simulink model "eVTOL_System"  (R2024b)
settings: Solver=FixedStepAuto  StartTime=0.0  StopTime=inf  RelTol=1e-3
undefined symbols (not defined in the file): airspeed, Battery, BCE12, BCE_Set_init, BMS_Controller_State, C, Cell10_P, Cell11_P, Cell12_P, Cell13_P, Cell14_P, Cell15_P, Cell16_P, Cell17_P, Cell18_P, Cell19_P, Cell1_N, Cell1_P, Cell20_P, Cell21_P, Cell22_P, Cell23_P, Cell24_P, Cell2_P, Cell3_P, Cell4_P, Cell5_P, Cell6_P, Cell7_P, Cell8_P, Cell9_P, Charging_State, CityMission, control, controlParams, ControlSampleTime, CriticalTiltAngle, currentFactor, CV_Gain, ddx, ddy, ddz, Device_01, Device_02, DiscIntNeverNeededParam, dx, dy, dz, Earth, env, F, F28379D_ADC_MaxCount, F28379D_ADC_Vmax, FixedWingMission, flightState, Foc_Ki_IxTcpu, Foc_Ki_S, Foc_Kp_I, Foc_Kp_S, fractalcoef ... (+68)
libraries: fl_lib x1115, nesl_utility x617, slrealtimeethercatlib x217, simulink x130, canmsglib x101, speedgoatlib_IO611_obsolete x91, slpidlib x49, mcbcontrolslib x44, slrealtimeutilitieslib x35, speedgoatlib_hdlCoder_IO3xx x31, dspstat3 x24, mcbpositiondecoderlib x12
(part 7 of 31)

== system eVTOL_System/Flight Controller/Autopilot/Fixed Wing Controller/Fixed Wing Controller Simulation ==
  note: Attitude Controller
  note: Lateral Guidance
  note: Airspeed-Altitude Controller
  note: Visualization
  In Bus Element14 : Inport  PortName=States  Element=Xe
  In Bus Element32 : Inport  PortName=States  Element=Xe
  In Bus Element15 : Inport  PortName=States  Element=course
  In Bus Element17 : Inport  PortName=States  Element=pqr
  In Bus Element{5,22..23,29} (4 alike) : Inport  PortName=States  Element=airspeed
  In Bus Element19 : Inport  PortName=States  Element=ypr
  In Bus Element27 : Inport  PortName=States  Element=ypr
  In Bus Element16 : Inport  PortName=States  Element=gndspeed
  In Bus Element26 : Inport  PortName=States  Element=Euler
  In Bus Element20 : Inport  PortName=States  Element=Ve_ground
  In Bus Element11 : Inport  Port=2  PortName=Control Mode  Element=lateralGuidance
  In Bus Element12 : Inport  Port=2  PortName=Control Mode  Element=airspeedAltitude
  In Bus Element13 : Inport  Port=2  PortName=Control Mode  Element=attitude
  In Bus Element1 : Inport  Port=3  PortName=AAC SP  Element=airspeed
  In Bus Element24 : Inport  Port=3  PortName=AAC SP  Element=airspeed
  In Bus Element2 : Inport  Port=3  PortName=AAC SP  Element=altitude
  In Bus Element33 : Inport  Port=3  PortName=AAC SP  Element=altitude
  In Bus Element18 : Inport  Port=3  PortName=AAC SP  Element=L1
  In Bus Element21 : Inport  Port=3  PortName=AAC SP  Element=course
  In Bus Element3 : Inport  Port=3  PortName=AAC SP  Element=course
  In Bus Element4 : Inport  Port=4  PortName=FixedWingSP  Element=yaw
  In Bus Element28 : Inport  Port=4  PortName=FixedWingSP  Element=yaw
  In Bus Element9 : Inport  Port=4  PortName=FixedWingSP  Element=pitch
  In Bus Element10 : Inport  Port=4  PortName=FixedWingSP  Element=roll
  In Bus Element8 : Inport  Port=4  PortName=FixedWingSP  Element=airspeed
  In Bus Element : Inport  Port=5  PortName=AERT  Element=aileron
  In Bus Element6 : Inport  Port=5  PortName=AERT  Element=elevator
  In Bus Element7 : Inport  Port=5  PortName=AERT  Element=rudder
  AER from Path Manager : Subsystem  TreatAsAtomicUnit=on
  Actuator dT Merge : Merge
  Airspeed Altitude Scope : Scope  NumInputPorts=2
  Airspeed-Altitude Controller : Subsystem
  Attitude Controller : Subsystem
  Demux : Demux  Outputs=3
  Demux1 : Demux  Outputs=3
  Gain1 : Gain  Gain=-1
  Lateral Guidance Logic : Subsystem
  Merge : Merge
  Mux : Mux  Inputs=3
  Mux1 : Mux  Inputs=3
  Mux{2..6} (5 alike) : Mux  Inputs=2
  NOT : Logic  Operator=NOT  IconShape=distinctive  AllPortsSameDT=off  OutDataTypeStr=boolean
  NOT1 : Logic  Operator=NOT  IconShape=distinctive  AllPortsSameDT=off  OutDataTypeStr=boolean
  NOT2 : Logic  Operator=NOT  IconShape=distinctive  AllPortsSameDT=off  OutDataTypeStr=boolean
  Pitch SP Merge : Merge
  "Pitch, Airspeed SP from Controller" : Subsystem  TreatAsAtomicUnit=on
  Roll SP Merge : Merge
  Roll SP from Path Manager : Subsystem  TreatAsAtomicUnit=on
  Selector1 : Selector  InputPortWidth=3  IndexOptions=Index vector (dialog)  Indices=[3]  OutputSizes=1
  Subsystem2 : Subsystem
  YPR Scope : Scope  NumInputPorts=3
  Bus Element Out : Outport  PortName=Actuator  Element=dA
  Out Bus Element : Outport  PortName=Actuator  Element=dE
  Out Bus Element1 : Outport  PortName=Actuator  Element=dR
  Out Bus Element2 : Outport  PortName=Actuator  Element=dT
  wires:
  [PitchSP] -> Mux2/1  "ref"
  In Bus Element24/1 -> Mux5/1
  Mux6/1 -> Airspeed Altitude Scope/2  "Altitude Tracking"
  Pitch SP Merge/1 -> Mux/2, [PitchSP]
  Demux/2 -> Out Bus Element/1
  Airspeed-Altitude Controller/1(Pitch SP) -> Pitch SP Merge/1
  In Bus Element18/1 -> Lateral Guidance Logic/2(L1 Distance)
  In Bus Element1/1 -> Airspeed-Altitude Controller/1(Airspeed SP)
  In Bus Element17/1 -> Subsystem2/2(pqr)
  Demux1/3 -> Mux3/2
  Demux1/1 -> Mux4/2
  Actuator dT Merge/1 -> Out Bus Element2/1
  In Bus Element26/1 -> Subsystem2/1(Euler)
  In Bus Element11/1 -> Lateral Guidance Logic/Enable, NOT/1
  Subsystem2/1(Euler Rate) -> Attitude Controller/3(Ang Rate)
  In Bus Element13/1 -> NOT2/1, Attitude Controller/Enable
  In Bus Element3/1 -> Lateral Guidance Logic/1(Course SP)
  In Bus Element22/1 -> Attitude Controller/4(Airspeed)
  Demux/3 -> Out Bus Element1/1
  Roll SP from Path Manager/1(Out1) -> Roll SP Merge/2
  In Bus Element4/1 -> Mux/1
  In Bus Element14/1 -> Airspeed-Altitude Controller/5(xyz)
  In Bus Element15/1 -> Lateral Guidance Logic/3(course)
  In Bus Element27/1 -> Demux1/1
  In Bus Element6/1 -> Mux1/2
  Mux1/1 -> AER from Path Manager/1(In1)
  Airspeed-Altitude Controller/2(Throttle) -> Actuator dT Merge/1
  "Pitch, Airspeed SP from Controller"/1(Pitch SP) -> Pitch SP Merge/2
  In Bus Element16/1 -> Lateral Guidance Logic/4(gndspeed)
  "Pitch, Airspeed SP from Controller"/2(Throttle) -> Actuator dT Merge/2
  In Bus Element/1 -> Mux1/1
  In Bus Element2/1 -> Airspeed-Altitude Controller/2(Altitude SP)
  In Bus Element7/1 -> Mux1/3
  In Bus Element9/1 -> "Pitch, Airspeed SP from Controller"/1(Pitch SP In)
  Merge/1 -> Demux/1
  In Bus Element10/1 -> Roll SP from Path Manager/1(In1)
  Mux/1 -> Attitude Controller/1(YPR SP)
  Attitude Controller/1(AER) -> Merge/1
  Demux1/2 -> Mux2/2
  NOT1/1 -> "Pitch, Airspeed SP from Controller"/Enable
  Gain1/1 -> Mux6/2
  In Bus Element8/1 -> "Pitch, Airspeed SP from Controller"/2(Airspeed SP)
  In Bus Element33/1 -> Mux6/1  "REF"
  In Bus Element20/1 -> Airspeed-Altitude Controller/6(vxyz)
  Mux3/1 -> YPR Scope/3  "Roll Tracking"
  Selector1/1 -> Gain1/1
  In Bus Element19/1 -> Attitude Controller/2(ypr)
  In Bus Element32/1 -> Selector1/1
  NOT2/1 -> AER from Path Manager/Enable
  In Bus Element23/1 -> "Pitch, Airspeed SP from Controller"/3(Airspeed)
  In Bus Element29/1 -> Mux5/2
  Lateral Guidance Logic/1(Roll SP) -> Roll SP Merge/1
  In Bus Element28/1 -> Mux4/1
  NOT/1 -> Roll SP from Path Manager/Enable
  AER from Path Manager/1(Out1) -> Merge/2
  In Bus Element5/1 -> Airspeed-Altitude Controller/4(Airspeed)
  Demux/1 -> Bus Element Out/1
  In Bus Element21/1 -> Airspeed-Altitude Controller/3(Climb Rate SP)
  Mux5/1 -> Airspeed Altitude Scope/1  "Airspeed Tracking"
  Mux2/1 -> YPR Scope/2  "Pitch Tracking"
  Roll SP Merge/1 -> [RollSP], Mux/3
  In Bus Element12/1 -> Airspeed-Altitude Controller/Enable, NOT1/1
  [RollSP] -> Mux3/1  "ref"
  Mux4/1 -> YPR Scope/1  "Yaw Tracking"

== system eVTOL_System/Flight Controller/Autopilot/Fixed Wing Controller/Fixed Wing Controller Tuning ==
  note: Visualization
  note: Attitude Controller
  note: Airspeed-Altitude Controller
  note: Lateral Guidance
  In Bus Element14 : Inport  PortName=States  Element=Xe
  In Bus Element32 : Inport  PortName=States  Element=Xe
  In Bus Element15 : Inport  PortName=States  Element=course
  In Bus Element17 : Inport  PortName=States  Element=pqr
  In Bus Element{5,22..23,29} (4 alike) : Inport  PortName=States  Element=airspeed
  In Bus Element19 : Inport  PortName=States  Element=ypr
  In Bus Element27 : Inport  PortName=States  Element=ypr
  In Bus Element16 : Inport  PortName=States  Element=gndspeed
  In Bus Element26 : Inport  PortName=States  Element=Euler
  In Bus Element20 : Inport  PortName=States  Element=Ve_ground
  In Bus Element11 : Inport  Port=2  PortName=Control Mode  Element=lateralGuidance
  In Bus Element12 : Inport  Port=2  PortName=Control Mode  Element=airspeedAltitude
  In Bus Element13 : Inport  Port=2  PortName=Control Mode  Element=attitude
  In Bus Element1 : Inport  Port=3  PortName=AAC SP  Element=airspeed
  In Bus Element24 : Inport  Port=3  PortName=AAC SP  Element=airspeed
  In Bus Element2 : Inport  Port=3  PortName=AAC SP  Element=altitude
  In Bus Element33 : Inport  Port=3  PortName=AAC SP  Element=altitude
  In Bus Element18 : Inport  Port=3  PortName=AAC SP  Element=L1
  In Bus Element21 : Inport  Port=3  PortName=AAC SP  Element=course
  In Bus Element3 : Inport  Port=3  PortName=AAC SP  Element=course
  In Bus Element4 : Inport  Port=4  PortName=FixedWingSP  Element=yaw
  In Bus Element28 : Inport  Port=4  PortName=FixedWingSP  Element=yaw
  In Bus Element9 : Inport  Port=4  PortName=FixedWingSP  Element=pitch
  In Bus Element10 : Inport  Port=4  PortName=FixedWingSP  Element=roll
  In Bus Element8 : Inport  Port=4  PortName=FixedWingSP  Element=airspeed
  In Bus Element : Inport  Port=5  PortName=AERT  Element=aileron
  In Bus Element6 : Inport  Port=5  PortName=AERT  Element=elevator
  In Bus Element7 : Inport  Port=5  PortName=AERT  Element=rudder
  AER Switch : Switch  Criteria=u2 > Threshold  SaturateOnIntegerOverflow=off  InputSameDT=off
  AER from Path Manager : Subsystem  TreatAsAtomicUnit=on
  Actuator dT Switch : Switch  Criteria=u2 > Threshold  SaturateOnIntegerOverflow=off  InputSameDT=off
  Airspeed Altitude Scope : Scope  NumInputPorts=2
  Airspeed-Altitude Controller : Subsystem
  Attitude Controller : Subsystem
  Demux : Demux  Outputs=3
  Demux1 : Demux  Outputs=3
  Gain : Gain  Gain=-1
  Lateral Guidance Logic : Subsystem
  Mux : Mux  Inputs=3
  Mux1 : Mux  Inputs=3
  Mux{2..6} (5 alike) : Mux  Inputs=2
  NOT : Logic  Operator=NOT  IconShape=distinctive  AllPortsSameDT=off  OutDataTypeStr=boolean
  NOT1 : Logic  Operator=NOT  IconShape=distinctive  AllPortsSameDT=off  OutDataTypeStr=boolean
  NOT2 : Logic  Operator=NOT  IconShape=distinctive  AllPortsSameDT=off  OutDataTypeStr=boolean
  Pitch SP Switch : Switch  Criteria=u2 > Threshold  SaturateOnIntegerOverflow=off  InputSameDT=off
  "Pitch, Airspeed SP from Controller" : Subsystem  TreatAsAtomicUnit=on
  Roll SP Switch : Switch  Criteria=u2 > Threshold  SaturateOnIntegerOverflow=off  InputSameDT=off
  Roll SP from Path Manager : Subsystem  TreatAsAtomicUnit=on
  Selector1 : Selector  InputPortWidth=3  IndexOptions=Index vector (dialog)  Indices=[3]  OutputSizes=1
  Subsystem2 : Subsystem
  YPR Scope : Scope  NumInputPorts=3
  Bus Element Out : Outport  PortName=Actuator  Element=dA
  Out Bus Element : Outport  PortName=Actuator  Element=dE
  Out Bus Element1 : Outport  PortName=Actuator  Element=dR
  Out Bus Element2 : Outport  PortName=Actuator  Element=dT
  wires:
  Mux/1 -> Attitude Controller/1(YPR SP)
  Attitude Controller/1(AER) -> AER Switch/1
  AER Switch/1 -> Demux/1
  Demux/1 -> Bus Element Out/1
  NOT/1 -> Roll SP from Path Manager/Enable
  Lateral Guidance Logic/1(Roll SP) -> Roll SP Switch/1
  Roll SP from Path Manager/1(Out1) -> Roll SP Switch/3
  NOT1/1 -> "Pitch, Airspeed SP from Controller"/Enable
  In Bus Element8/1 -> "Pitch, Airspeed SP from Controller"/2(Airspeed SP)
  "Pitch, Airspeed SP from Controller"/1(Pitch SP) -> Pitch SP Switch/3
  Airspeed-Altitude Controller/2(Throttle) -> Actuator dT Switch/1
  "Pitch, Airspeed SP from Controller"/2(Throttle) -> Actuator dT Switch/3
  Mux1/1 -> AER from Path Manager/1(In1)
  AER from Path Manager/1(Out1) -> AER Switch/3
  NOT2/1 -> AER from Path Manager/Enable
  In Bus Element/1 -> Mux1/1
  In Bus Element6/1 -> Mux1/2
  In Bus Element7/1 -> Mux1/3
  In Bus Element9/1 -> "Pitch, Airspeed SP from Controller"/1(Pitch SP In)
  In Bus Element10/1 -> Roll SP from Path Manager/1(In1)
  In Bus Element11/1 -> Roll SP Switch/2, Lateral Guidance Logic/Enable, NOT/1
  In Bus Element18/1 -> Lateral Guidance Logic/2(L1 Distance)
  In Bus Element14/1 -> Airspeed-Altitude Controller/5(xyz)
  In Bus Element19/1 -> Attitude Controller/2(ypr)
  In Bus Element16/1 -> Lateral Guidance Logic/4(gndspeed)
  In Bus Element5/1 -> Airspeed-Altitude Controller/4(Airspeed)
  In Bus Element12/1 -> Actuator dT Switch/2, Pitch SP Switch/2, Airspeed-Altitude Controller/Enable, NOT1/1
  In Bus Element2/1 -> Airspeed-Altitude Controller/2(Altitude SP)
  Roll SP Switch/1 -> Mux/3, [RollSP]
  In Bus Element15/1 -> Lateral Guidance Logic/3(course)
  Demux/3 -> Out Bus Element1/1
  In Bus Element13/1 -> NOT2/1, AER Switch/2, Attitude Controller/Enable
  In Bus Element4/1 -> Mux/1
  In Bus Element22/1 -> Attitude Controller/4(Airspeed)
  In Bus Element3/1 -> Lateral Guidance Logic/1(Course SP)
  In Bus Element1/1 -> Airspeed-Altitude Controller/1(Airspeed SP)
  In Bus Element20/1 -> Airspeed-Altitude Controller/6(vxyz)
  In Bus Element21/1 -> Airspeed-Altitude Controller/3(Climb Rate SP)
  In Bus Element23/1 -> "Pitch, Airspeed SP from Controller"/3(Airspeed)
  In Bus Element27/1 -> Demux1/1
  Demux1/1 -> Mux4/2
  Demux1/2 -> Mux2/2
  Demux1/3 -> Mux3/2
  In Bus Element17/1 -> Subsystem2/2(pqr)
  In Bus Element26/1 -> Subsystem2/1(Euler)
  Subsystem2/1(Euler Rate) -> Attitude Controller/3(Ang Rate)
  Actuator dT Switch/1 -> Out Bus Element2/1
  Demux/2 -> Out Bus Element/1
  Pitch SP Switch/1 -> [PitchSP], Mux/2
  Airspeed-Altitude Controller/1(Pitch SP) -> Pitch SP Switch/1
  [PitchSP] -> Mux2/1  "ref"
  In Bus Element28/1 -> Mux4/1
  [RollSP] -> Mux3/1  "ref"
  Mux4/1 -> YPR Scope/1  "Yaw Tracking"
  Mux2/1 -> YPR Scope/2  "Pitch Tracking"
  Mux3/1 -> YPR Scope/3  "Roll Tracking"
  Mux5/1 -> Airspeed Altitude Scope/1  "Airspeed Tracking"
  Mux6/1 -> Airspeed Altitude Scope/2  "Altitude Tracking"
  In Bus Element24/1 -> Mux5/1
  In Bus Element29/1 -> Mux5/2
  In Bus Element32/1 -> Selector1/1
  Selector1/1 -> Gain/1
  Gain/1 -> Mux6/2
  In Bus Element33/1 -> Mux6/1  "REF"

== system eVTOL_System/Flight Controller/Autopilot/Multicopter Controller/Altitude Control ==
  note: Maintain altitude previously set when in transition
  Z ref : Inport
  States : Inport  Port=2
  InTransition : Inport  Port=3
  Bus Selector : BusSelector  OutputSignals=Xe,Ve
  Constant : Constant  Value=0
  Gain1 : Gain  Gain=controlParams.D_Z
  NOT : Logic  Operator=NOT  IconShape=distinctive  AllPortsSameDT=off  OutDataTypeStr=boolean
  PID Controller : slpidlib/PID Controller  Controller=P  Form=Parallel  TimeDomain=Discrete-time  UseExternalTs=off  SampleTime=-1  IntegratorMethod=Forward Euler  FilterMethod=Forward Euler  ControllerParametersSource=internal  P=controlParams.P_Z  I=controlParams.I_Z  UseKiTs=off  D=controlParams.D_Z  UseExternalDerivativeSource=off  N=controlParams.N_Z  UseFilter=on  TunerSelectOption=Transfer Function Based (PID Tuner App)  InitialConditionSource=internal  InitialConditionForIntegrator=0  InitialConditionForFilter=0  DifferentiatorICPrevScaledInput=0  ExternalReset=none  TrackingMode=off  Kt=1  LimitOutput=off  SatLimitsSource=internal  UpperSaturationLimit=inf  LowerSaturationLimit=-inf  LinearizeAsGain=on  AntiWindupMode=none  Kb=1  LimitIntegrator=off  UpperIntegratorSaturationLimit=inf  LowerIntegratorSaturationLimit=-inf  POutMin=[]  POutMax=[]  IOutMin=[]  IOutMax=[]  DOutMin=[]  DOutMax=[]  NOutMin=[]  NOutMax=[]  SumOutMin=[]  SumOutMax=[]  SaturationOutMin=[]  SaturationOutMax=[]  PParamMin=[]  PParamMax=[]  IParamMin=[]  IParamMax=[]  DParamMin=[]  DParamMax=[]  NParamMin=[]  NParamMax=[]  KbParamMin=[]  KbParamMax=[]  KtParamMin=[]  KtParamMax=[]  KbOutMin=[]  KbOutMax=[]  KtOutMin=[]  KtOutMax=[]  IntegratorOutMin=[]  IntegratorOutMax=[]  FilterOutMin=[]  FilterOutMax=[]  SumI1OutMin=[]  SumI1OutMax=[]  SumI2OutMin=[]  SumI2OutMax=[]  SumI3OutMin=[]  SumI3OutMax=[]  SumI4OutMin=[]  SumI4OutMax=[]  SumDOutMin=[]  SumDOutMax=[]  DifferentiatorOutMin=[]  DifferentiatorOutMax=[]  FilterDiffOutCoefMin=[]  FilterDiffOutCoefMax=[]  ReciprocalOutMin=[]  ReciprocalOutMax=[]  SumDenOutMin=[]  SumDenOutMax=[]  SumNumOutMin=[]  SumNumOutMax=[]  DivideOutMin=[]  DivideOutMax=[]  UdiffTsProdOutMin=[]  UdiffTsProdOutMax=[]  NTsProdOutMin=[]  NTsProdOutMax=[]  UintegralTsProdOutMin=[]  UintegralTsProdOutMax=[]  UngainTsProdOutMin=[]  UngainTsProdOutMax=[]  ClampingZeroOutDataTypeStr=Inherit: Inherit via back propagation  ClampingZeroOutMin=[]  ClampingZeroOutMax=[]  FilterDenConstantOutDataTypeStr=Inherit: Inherit via back propagation  FilterDenConstantOutMin=[]  FilterDenConstantOutMax=[]  PCopyOutDataTypeStr=Inherit: Inherit via back propagation  PCopyOutMin=[]  PCopyOutMax=[]  NCopyOutDataTypeStr=Inherit: Inherit via back propagation  NCopyOutMin=[]  NCopyOutMax=[]  IntegratorContinuousStateAttributes=''  IntegratorStateMustResolveToSignalObject=off  IntegratorRTWStateStorageClass=Auto  FilterContinuousStateAttributes=''  FilterStateMustResolveToSignalObject=off  FilterRTWStateStorageClass=Auto  ParallelPVariant=InternalParameters  IdealPVariant=Disabled  IVariant=Disabled  DVariant=Disabled  IntegratorVariant=Disabled  SatVariant=Disabled  AWVariant=Disabled  PCopyVariant=Disabled  TRVariant=Disabled  FdbkBlocksVariant=Forward  IdealPFdbkVariant=Disabled  SatFdbkVariant=Disabled  DerivativeFilterVariant=Disabled  NVariant=Disabled  NCopyVariant=Disabled_SignalSpec  FilterICVariant=Disabled  IntegratorICVariant=Disabled  ExternalResetVariant=Disabled  TRSumVariant=Passthrough  SumFdbkVariant=Disabled  SumVariant=Passthrough_P  TsampFilterVariant=InternalTs  TsampNgainVariant=Passthrough  TsampIntegralVariant=Disabled_SignalSpec  ExternalSaturationOutDataTypeStr=Inherit: Same as second input  DerivativeSourceVariant=Disabled  PreIntVariant=InternalPreInt
  PID Controller1 : slpidlib/PID Controller  Controller=PID  Form=Parallel  TimeDomain=Discrete-time  UseExternalTs=off  SampleTime=-1  IntegratorMethod=Forward Euler  FilterMethod=Forward Euler  ControllerParametersSource=internal  P=controlParams.P_VZ  I=controlParams.I_Z  UseKiTs=off  D=controlParams.D_VZ  UseExternalDerivativeSource=off  N=controlParams.N_VZ  UseFilter=on  TunerSelectOption=Transfer Function Based (PID Tuner App)  InitialConditionSource=internal  InitialConditionForIntegrator=0  InitialConditionForFilter=0  DifferentiatorICPrevScaledInput=0  ExternalReset=none  TrackingMode=off  Kt=1  LimitOutput=off  SatLimitsSource=internal  UpperSaturationLimit=inf  LowerSaturationLimit=-inf  LinearizeAsGain=on  AntiWindupMode=none  Kb=1  LimitIntegrator=off  UpperIntegratorSaturationLimit=inf  LowerIntegratorSaturationLimit=-inf  POutMin=[]  POutMax=[]  IOutMin=[]  IOutMax=[]  DOutMin=[]  DOutMax=[]  NOutMin=[]  NOutMax=[]  SumOutMin=[]  SumOutMax=[]  SaturationOutMin=[]  SaturationOutMax=[]  PParamMin=[]  PParamMax=[]  IParamMin=[]  IParamMax=[]  DParamMin=[]  DParamMax=[]  NParamMin=[]  NParamMax=[]  KbParamMin=[]  KbParamMax=[]  KtParamMin=[]  KtParamMax=[]  KbOutMin=[]  KbOutMax=[]  KtOutMin=[]  KtOutMax=[]  IntegratorOutMin=[]  IntegratorOutMax=[]  FilterOutMin=[]  FilterOutMax=[]  SumI1OutMin=[]  SumI1OutMax=[]  SumI2OutMin=[]  SumI2OutMax=[]  SumI3OutMin=[]  SumI3OutMax=[]  SumI4OutMin=[]  SumI4OutMax=[]  SumDOutMin=[]  SumDOutMax=[]  DifferentiatorOutMin=[]  DifferentiatorOutMax=[]  FilterDiffOutCoefMin=[]  FilterDiffOutCoefMax=[]  ReciprocalOutMin=[]  ReciprocalOutMax=[]  SumDenOutMin=[]  SumDenOutMax=[]  SumNumOutMin=[]  SumNumOutMax=[]  DivideOutMin=[]  DivideOutMax=[]  UdiffTsProdOutMin=[]  UdiffTsProdOutMax=[]  NTsProdOutMin=[]  NTsProdOutMax=[]  UintegralTsProdOutMin=[]  UintegralTsProdOutMax=[]  UngainTsProdOutMin=[]  UngainTsProdOutMax=[]  ClampingZeroOutDataTypeStr=Inherit: Inherit via back propagation  ClampingZeroOutMin=[]  ClampingZeroOutMax=[]  FilterDenConstantOutDataTypeStr=Inherit: Inherit via back propagation  FilterDenConstantOutMin=[]  FilterDenConstantOutMax=[]  PCopyOutDataTypeStr=Inherit: Inherit via back propagation  PCopyOutMin=[]  PCopyOutMax=[]  NCopyOutDataTypeStr=Inherit: Inherit via back propagation  NCopyOutMin=[]  NCopyOutMax=[]  IntegratorContinuousStateAttributes=''  IntegratorStateMustResolveToSignalObject=off  IntegratorRTWStateStorageClass=Auto  FilterContinuousStateAttributes=''  FilterStateMustResolveToSignalObject=off  FilterRTWStateStorageClass=Auto  ParallelPVariant=InternalParameters  IdealPVariant=Disabled  IVariant=InternalParameters  DVariant=InternalParameters  IntegratorVariant=Discrete  SatVariant=Disabled  AWVariant=Passthrough  PCopyVariant=Disabled  TRVariant=Disabled  FdbkBlocksVariant=Forward  IdealPFdbkVariant=Disabled  SatFdbkVariant=Disabled  DerivativeFilterVariant=ForwardEulerFilter  NVariant=InternalParameters  NCopyVariant=Disabled  FilterICVariant=InternalICsFilter  IntegratorICVariant=InternalICs  ExternalResetVariant=Disabled  TRSumVariant=Passthrough  SumFdbkVariant=Disabled  SumVariant=Sum_PID  TsampFilterVariant=InternalTs  TsampNgainVariant=Passthrough  TsampIntegralVariant=Disabled_SignalSpec  ExternalSaturationOutDataTypeStr=Inherit: Same as second input  DerivativeSourceVariant=ErrorSignal  PreIntVariant=InternalPreInt
  Rate Limiter : RateLimiter  FallingSlewLimit=-1000  SampleTimeMode=inherited
  Selector : Selector  InputPortWidth=3  IndexOptions=Index vector (dialog)  Indices=[3]  OutputSizes=1
  Selector1 : Selector  InputPortWidth=3  IndexOptions=Index vector (dialog)  Indices=[3]  OutputSizes=1
  Sum : Sum  Inputs=|+-
  Sum1 : Sum  Inputs=|+-
  Sum2 : Sum  Inputs=|++
  Sum3 : Sum  Inputs=|--
  Switch : Switch  Criteria=u2 > Threshold  SaturateOnIntegerOverflow=off  InputSameDT=off
  Triggered Subsystem : Subsystem  TreatAsAtomicUnit=on
  commanded thrust : Outport
  wires:
  Sum/1 -> PID Controller/1
  Z ref/1 -> Switch/1  "Manual"
  States/1 -> Bus Selector/1
  InTransition/1 -> NOT/1, Triggered Subsystem/Trigger
  Switch/1 -> Rate Limiter/1  "Output"
  NOT/1 -> Switch/2
  Triggered Subsystem/1(Reference) -> Switch/3  "Stable"
  Selector/1 -> Sum/2, Triggered Subsystem/1(AltHold)
  Bus Selector/1 -> Selector/1  "<Xe>"
  Bus Selector/2 -> Selector1/1  "<Ve>"
  PID Controller/1 -> Sum2/1
  Selector1/1 -> Sum1/2, Gain1/1
  Gain1/1 -> Sum3/2
  Sum2/1 -> Sum1/1
  Sum1/1 -> PID Controller1/1
  Rate Limiter/1 -> Sum/1
  Sum3/1 -> Sum2/2
  PID Controller1/1 -> commanded thrust/1
  Constant/1 -> Sum3/1

== system eVTOL_System/Flight Controller/Autopilot/Multicopter Controller/Attitude Control ==
  Ref Attitude : Inport
  States : Inport  Port=2
  inTransition : Inport  Port=3
  Attitude Control : Subsystem  VariantControl=AttitudeControl==0
  Derivative Gain : Subsystem  VariantControl=AttitudeControl==1
  Roll torque cmd : Outport
  Pitch torque Cmd : Outport  Port=2
  Yaw torque Cmd : Outport  Port=3

== system eVTOL_System/Flight Controller/Autopilot/Multicopter Controller/Attitude Stabilization ==
  note: Level Tiltrotor when in transition.
  Enable : EnablePort
  Constant : Constant  Value=0
  Constant1 : Constant  Value=0
  Tilt Cmd : Outport
  Roll Cmd : Outport  Port=2
  wires:
  Constant/1 -> Tilt Cmd/1
  Constant1/1 -> Roll Cmd/1

== system eVTOL_System/Flight Controller/Autopilot/Multicopter Controller/Horizontal Position Control ==
  note: Forward Motion is controlled using Tilt.
      | Lateral Motion occurs using roll.
  XRef : Inport
  YRef : Inport  Port=2
  States : Inport  Port=3
  Enable : EnablePort
  Saturation : Saturate  UpperLimit=0.4  LowerLimit=-0.4
  XY Controller : Subsystem
  Roll Cmd : Outport
  Tilt Cmd : Outport  Port=2
  wires:
  XRef/1 -> XY Controller/1(X_ref)
  YRef/1 -> XY Controller/2(Y_ref)
  States/1 -> XY Controller/3(States)
  XY Controller/1(Forward cmd) -> Tilt Cmd/1
  XY Controller/2(Sideward Cmd) -> Saturation/1
  Saturation/1 -> Roll Cmd/1

== system eVTOL_System/Flight Controller/Autopilot/Multicopter Controller/Organize Inputs ==
  forward command : Inport
  commanded phi torque : Inport  Port=2
  commanded theta torque : Inport  Port=3
  commanded psi torque : Inport  Port=4
  commanded thrust : Inport  Port=5
  Out Bus Element : Outport  PortName=MixerCommands  Element=w_phi
  Out Bus Element1 : Outport  PortName=MixerCommands  Element=w_theta
  Out Bus Element2 : Outport  PortName=MixerCommands  Element=l_psi
  Out Bus Element3 : Outport  PortName=MixerCommands  Element=w_z
  Out Bus Element4 : Outport  PortName=MixerCommands  Element=l_x
  tag scope: w_phi=global, w_psi=global, w_theta=global, w_tilt=global, w_z=global
  wires:
  commanded theta torque/1 -> Out Bus Element1/1, [w_theta]  "theta"
  commanded psi torque/1 -> Out Bus Element2/1, [w_psi]  "psi"
  commanded thrust/1 -> Out Bus Element3/1, [w_z]  "thrust"
  forward command/1 -> Out Bus Element4/1, [w_tilt]  "tilt"
  commanded phi torque/1 -> Out Bus Element/1, [w_phi]  "phi"

== system eVTOL_System/Flight Controller/Autopilot/Multicopter Controller/Subsystem ==
  inTransition : Inport
  States : Inport  Port=2
  Reference : Inport  Port=3
  Bus Selector : BusSelector  OutputSignals=ypr
  Bus Selector1 : BusSelector  OutputSignals=ypr,Euler
  NOT : Logic  Operator=NOT  IconShape=distinctive  AllPortsSameDT=off  OutDataTypeStr=boolean
  Scope{,1..3} (4 alike) : Scope
  Selector : Selector  InputPortWidth=3  IndexOptions=Index vector (dialog)  Indices=[1]  OutputSizes=1
  Switch : Switch  Criteria=u2 > Threshold  SaturateOnIntegerOverflow=off  InputSameDT=off
  Triggered Subsystem : Subsystem  TreatAsAtomicUnit=on
  Yaw Reference : Outport
  wires:
  inTransition/1 -> Triggered Subsystem/Trigger, NOT/1
  States/1 -> Bus Selector1/1, Bus Selector/1
  Bus Selector/1 -> Selector/1  "<ypr>"
  Selector/1 -> Triggered Subsystem/1(YawHold)
  NOT/1 -> Switch/2
  Triggered Subsystem/1(Reference) -> Switch/3, Scope1/1  "Stable"
  Switch/1 -> Scope/1, Yaw Reference/1
  Bus Selector1/1 -> Scope2/1  "<ypr>"
  Bus Selector1/2 -> Scope3/1  "<Euler>"
  Reference/1 -> Switch/1

== system eVTOL_System/Flight Controller/Autopilot/Tilt Scheduler/Back Transition Scheduler ==
  Tilt Schedule : Inport
  FlightMode : Inport  Port=2
  States : Inport  Port=3
  Add : Sum  Inputs=+-
  Bus Selector : BusSelector  OutputSignals=Vb
  Constant1 : Constant  Value=flightState.BackTransition
  Constant6 : Constant  Value=0
  Equal1 : RelationalOperator  Operator===  OutDataTypeStr=boolean  RndMeth=Simplest  InputSameDT=off
  Saturation : Saturate  UpperLimit=pi/4  LowerLimit=-pi/4
  Selector : Selector  InputPortWidth=3  IndexOptions=Index vector (dialog)  Indices=[1]  OutputSizes=1
  Switch2 : Switch  Threshold=1  SaturateOnIntegerOverflow=off  InputSameDT=off
  Vx Controller : slpidlib/PID Controller  Controller=P  Form=Parallel  TimeDomain=Discrete-time  UseExternalTs=off  SampleTime=0.005  IntegratorMethod=Forward Euler  FilterMethod=Forward Euler  ControllerParametersSource=internal  P=controlParams.P_BACK  I=0  UseKiTs=off  D=0.0379422021775223  UseExternalDerivativeSource=off  N=1.96946409823213  UseFilter=on  TunerSelectOption=Transfer Function Based (PID Tuner App)  InitialConditionSource=internal  InitialConditionForIntegrator=0  InitialConditionForFilter=0  DifferentiatorICPrevScaledInput=0  ExternalReset=none  TrackingMode=off  Kt=1  LimitOutput=off  SatLimitsSource=internal  UpperSaturationLimit=inf  LowerSaturationLimit=-inf  LinearizeAsGain=on  AntiWindupMode=none  Kb=1  LimitIntegrator=off  UpperIntegratorSaturationLimit=inf  LowerIntegratorSaturationLimit=-inf  POutMin=[]  POutMax=[]  IOutMin=[]  IOutMax=[]  DOutMin=[]  DOutMax=[]  NOutMin=[]  NOutMax=[]  SumOutMin=[]  SumOutMax=[]  SaturationOutMin=[]  SaturationOutMax=[]  PParamMin=[]  PParamMax=[]  IParamMin=[]  IParamMax=[]  DParamMin=[]  DParamMax=[]  NParamMin=[]  NParamMax=[]  KbParamMin=[]  KbParamMax=[]  KtParamMin=[]  KtParamMax=[]  KbOutMin=[]  KbOutMax=[]  KtOutMin=[]  KtOutMax=[]  IntegratorOutMin=[]  IntegratorOutMax=[]  FilterOutMin=[]  FilterOutMax=[]  SumI1OutMin=[]  SumI1OutMax=[]  SumI2OutMin=[]  SumI2OutMax=[]  SumI3OutMin=[]  SumI3OutMax=[]  SumI4OutMin=[]  SumI4OutMax=[]  SumDOutMin=[]  SumDOutMax=[]  DifferentiatorOutMin=[]  DifferentiatorOutMax=[]  FilterDiffOutCoefMin=[]  FilterDiffOutCoefMax=[]  ReciprocalOutMin=[]  ReciprocalOutMax=[]  SumDenOutMin=[]  SumDenOutMax=[]  SumNumOutMin=[]  SumNumOutMax=[]  DivideOutMin=[]  DivideOutMax=[]  UdiffTsProdOutMin=[]  UdiffTsProdOutMax=[]  NTsProdOutMin=[]  NTsProdOutMax=[]  UintegralTsProdOutMin=[]  UintegralTsProdOutMax=[]  UngainTsProdOutMin=[]  UngainTsProdOutMax=[]  ClampingZeroOutDataTypeStr=Inherit: Inherit via back propagation  ClampingZeroOutMin=[]  ClampingZeroOutMax=[]  FilterDenConstantOutDataTypeStr=Inherit: Inherit via back propagation  FilterDenConstantOutMin=[]  FilterDenConstantOutMax=[]  PCopyOutDataTypeStr=Inherit: Inherit via back propagation  PCopyOutMin=[]  PCopyOutMax=[]  NCopyOutDataTypeStr=Inherit: Inherit via back propagation  NCopyOutMin=[]  NCopyOutMax=[]  IntegratorContinuousStateAttributes=''  IntegratorStateMustResolveToSignalObject=off  IntegratorRTWStateStorageClass=Auto  FilterContinuousStateAttributes=''  FilterStateMustResolveToSignalObject=off  FilterRTWStateStorageClass=Auto  ParallelPVariant=InternalParameters  IdealPVariant=Disabled  IVariant=Disabled  DVariant=Disabled  IntegratorVariant=Disabled  SatVariant=Disabled  AWVariant=Disabled  PCopyVariant=Disabled  TRVariant=Disabled  FdbkBlocksVariant=Forward  IdealPFdbkVariant=Disabled  SatFdbkVariant=Disabled  DerivativeFilterVariant=Disabled  NVariant=Disabled  NCopyVariant=Disabled_SignalSpec  FilterICVariant=Disabled  IntegratorICVariant=Disabled  ExternalResetVariant=Disabled  TRSumVariant=Passthrough  SumFdbkVariant=Disabled  SumVariant=Passthrough_P  TsampFilterVariant=InternalTs  TsampNgainVariant=Passthrough  TsampIntegralVariant=Disabled_SignalSpec  ExternalSaturationOutDataTypeStr=Inherit: Same as second input  DerivativeSourceVariant=Disabled  PreIntVariant=InternalPreInt
  TiltAngle : Outport
  wires:
  States/1 -> Bus Selector/1
  Add/1 -> Vx Controller/1
  Equal1/1 -> Switch2/2
  Bus Selector/1 -> Selector/1  "<Vb>"
  FlightMode/1 -> Equal1/1
  Constant1/1 -> Equal1/2
  Constant6/1 -> Add/1
  Selector/1 -> Add/2
  Vx Controller/1 -> Saturation/1
  Saturation/1 -> Switch2/1
  Tilt Schedule/1 -> Switch2/3
  Switch2/1 -> TiltAngle/1

== system eVTOL_System/Flight Controller/Autopilot/Tilt Scheduler/Forward Transition Scheduler ==
  FlightMode : Inport
  Constant : Constant  Value=pi/2
  Constant2 : Constant  Value=0
  Constant3 : Constant  Value=CriticalTiltAngle
  Constant4 : Constant  Value=flightState.Transition
  Constant5 : Constant  Value=TiltScheduleRate
  Equal : RelationalOperator  Operator===  OutDataTypeStr=boolean  RndMeth=Simplest  InputSameDT=off
  Integrator : Integrator  ExternalReset=either  LimitOutput=on  UpperSaturationLimit=Inf  LowerSaturationLimit=0
  LessThanOrEqual : RelationalOperator  Operator=<=  OutDataTypeStr=boolean  RndMeth=Simplest  InputSameDT=off
  Switch : Switch  Criteria=u2 > Threshold  SaturateOnIntegerOverflow=off  InputSameDT=off
  Switch1 : Switch  Criteria=u2 > Threshold  SaturateOnIntegerOverflow=off  InputSameDT=off
  FlightState : Outport
  Tilt Schedule : Outport  Port=2
  tag scope: ModeFlag=global
  wires:
  FlightMode/1 -> FlightState/1, Equal/2
  [ModeFlag] -> Switch1/2, Integrator/2
  Integrator/1 -> Switch/1, LessThanOrEqual/1
  LessThanOrEqual/1 -> Switch/2
  Equal/1 -> [ModeFlag]
  Constant3/1 -> LessThanOrEqual/2
  Switch1/1 -> Integrator/1
  Constant5/1 -> Switch1/1
  Constant2/1 -> Switch1/3
  Constant4/1 -> Equal/1
  Constant/1 -> Switch/3
  Switch/1 -> Tilt Schedule/1

== system eVTOL_System/Flight Controller/Estimator/Estimation Filter/Airspeed Filter ==
  DiffPress : Inport
  rho : Inport  Port=2
  Constant : Constant  Value=0.5
  Divide : Product  Inputs=*/
  Product : Product
  Sqrt : Sqrt
  airspeed : Outport
  wires:
  Constant/1 -> Product/2
  rho/1 -> Product/1
  Product/1 -> Divide/2
  DiffPress/1 -> Divide/1
  Divide/1 -> Sqrt/1
  Sqrt/1 -> airspeed/1

== system eVTOL_System/Flight Controller/Estimator/Estimation Filter/LLA2Local ==
  LLA : Inport
  Constant1 : Constant  Value=0
  Demux1 : Demux  Outputs=2
  LLA to Flat Earth1 : aerolibtransform2/LLA to Flat Earth  units=Metric (MKS)  ptype=Earth (WGS84)  F=1/298.257223563  R=6378137  refPosPort=off  LL0=[0 0]  psi=0
  Xe : Outport
  wires:
  Constant1/1 -> LLA to Flat Earth1/3
  Demux1/1 -> LLA to Flat Earth1/1
  Demux1/2 -> LLA to Flat Earth1/2
  LLA to Flat Earth1/1 -> Xe/1  "Xe"
  LLA/1 -> Demux1/1

== system eVTOL_System/Flight Controller/Ground Control Station/Get Flight Mission/noQGC ==
  note: uavPathManagerBus type
  No Mission : Constant  Value=struct('mode',0,'position',[0 0 0]','params',[0;0;0;0]);  OutDataTypeStr=Bus: doubleUavPathManager
  Variant Source : VariantSource
  Waypoints : Constant  Value=FixedWingMission  OutDataTypeStr=Bus: doubleUavPathManager  SampleTime=-1
  Waypoints1 : Constant  Value=HoverMission  OutDataTypeStr=Bus: doubleUavPathManager  SampleTime=-1
  Waypoints2 : Constant  Value=TransitionMission  OutDataTypeStr=Bus: doubleUavPathManager  SampleTime=-1
  Waypoints3 : Constant  Value=CityMission  OutDataTypeStr=Bus: doubleUavPathManager  SampleTime=-1
  Mission : Outport
  wires:
  Waypoints/1 -> Variant Source/2
  Waypoints1/1 -> Variant Source/3
  Variant Source/1 -> Mission/1
  Waypoints2/1 -> Variant Source/4
  No Mission/1 -> Variant Source/1
  Waypoints3/1 -> Variant Source/5

== system eVTOL_System/Flight Controller/Guidance Test Bench/ControlType/Guidance Testbench ==
  Global Mission : Inport
  Aircraft States : Inport  Port=2
  Control Rate Transition : Subsystem
  Guidance Logic : Subsystem  VariantControl=guidanceType==1
  HoverCmds : Outport
  FixedWingSP : Outport  Port=2
  AACSP : Outport  Port=3
  ctrlMode : Outport  Port=4
  FlightMode : Outport  Port=5
  wires:
  Aircraft States/1 -> Guidance Logic/1(UAVState)
  Global Mission/1 -> Guidance Logic/2(GCSCommands)
  Guidance Logic/1(HoverGuidance) -> Control Rate Transition/1("1 ")
  Guidance Logic/2(FixedWingSP) -> Control Rate Transition/2(In2)
  Guidance Logic/3(AACSP) -> Control Rate Transition/3(In3)
  Guidance Logic/4(ctrlMode) -> Control Rate Transition/4(In4)
  Guidance Logic/5(FlightMode) -> Control Rate Transition/5(In5)
  Control Rate Transition/1(Out1) -> HoverCmds/1
  Control Rate Transition/2(Out2) -> FixedWingSP/1
  Control Rate Transition/3(Out3) -> AACSP/1
  Control Rate Transition/4(Out4) -> ctrlMode/1
  Control Rate Transition/5(Out5) -> FlightMode/1

== system eVTOL_System/Flight Controller/Guidance Test Bench/ControlType/Manual Control ==
  note: Change these parameters during simulation when using manual testbench mode.
  note: Commanded Altitude (m)
  note: Commanded Y (m)
  note: Fixed Wing Aerodynamics
  note: Commanded X (m)
  note: Fixed Wing
  note: Hover
  note: Flight Mode
  note: Transition
  note: Commanded Course
  note: Commanded Altitude
  note: Commanded Airspeed (m)
  note: Back Transition
  note: Fixed Wing Commands
  note: Hover Commands
  Global Mission : Inport
  Aircraft States : Inport  Port=2
  Command Interface : Subsystem
  Slider1 : SliderBlock  LabelPosition=Hide  ScaleMax=50  TickInterval=5
  Slider2 : SliderBlock  LabelPosition=Hide  ScaleMin=-30  ScaleMax=30  TickInterval=5
  Slider3 : SliderBlock  LabelPosition=Hide  ScaleMin=-30  ScaleMax=30  TickInterval=5
  Slider4 : SliderBlock  LabelPosition=Hide  ScaleMax=3  TickInterval=1
  Slider5 : SliderBlock  LabelPosition=Hide  ScaleMin=-30  ScaleMax=30  TickInterval=5
  Slider6 : SliderBlock  LabelPosition=Hide  ScaleMin=-100  TickInterval=10
  Slider7 : SliderBlock  LabelPosition=Hide  ScaleMin=10  ScaleMax=30  TickInterval=5
  Toggle Switch1 : ToggleSwitchBlock  LabelPosition=Hide
      settings: Values={{'Off', 'On'}, [0 1]}
  HoverCmds : Outport
  FixedWingSP : Outport  Port=2
  AACSP : Outport  Port=3
  ctrlMode : Outport  Port=4
  FlightMode : Outport  Port=5
  wires:
  Global Mission/1 -> Command Interface/1(Global Mission)
  Aircraft States/1 -> Command Interface/2(Aircraft States)
  Command Interface/1(ctrlMode) -> ctrlMode/1
  Command Interface/2(FixedWingSP) -> FixedWingSP/1
  Command Interface/3(AACSP) -> AACSP/1
  Command Interface/4(PositionCmds) -> HoverCmds/1
  Command Interface/5(FlightMode) -> FlightMode/1

== system eVTOL_System/Flight Controller/Guidance Test Bench/Reference Tracking /Fixed Wing Reference ==
  AAC Commands : Inport
  States : Inport  Port=2
  Bus Creator1 : BusCreator  Inputs=2
  Bus Creator2 : BusCreator  Inputs=3
  Bus Selector : BusSelector  OutputSignals=airspeed,Xe,course
  Bus Selector3 : BusSelector  OutputSignals=airspeed,altitude,course
  Gain : Gain  Gain=-1
  Mux1 : Mux  Inputs=3
  Selector : Selector  InputPortWidth=3  IndexOptions=Index vector (dialog)  Indices=3  OutputSizes=1
  To Workspace1 : ToWorkspace  VariableName=FixedWingCmdFdbk  SaveFormat=Structure With Time  SampleTime=-1
  wires:
  Selector/1 -> Gain/1
  Bus Selector3/1 -> Mux1/1  "<airspeed>"
  Bus Selector/1 -> Bus Creator2/1  "<airspeed>"
  Bus Selector3/2 -> Mux1/2  "<altitude>"
  Bus Selector/3 -> Bus Creator2/3  "<course>"
  Mux1/1 -> Bus Creator1/1
  Bus Creator1/1 -> To Workspace1/1
  Bus Selector3/3 -> Mux1/3  "<course>"
  Gain/1 -> Bus Creator2/2  "altitude"
  Bus Creator2/1 -> Bus Creator1/2
  AAC Commands/1 -> Bus Selector3/1
  Bus Selector/2 -> Selector/1  "<Xe>"
  States/1 -> Bus Selector/1

== system eVTOL_System/Flight Controller/Guidance Test Bench/Reference Tracking /Hover Reference ==
  Position Command : Inport
  Position Reference : Inport  Port=2
  Bus Creator : BusCreator  Inputs=2
  Bus Selector1 : BusSelector  OutputSignals=Xe  OutputAsBus=on
  Bus Selector2 : BusSelector  OutputSignals=X,Y,Z
  Mux : Mux  Inputs=3
  To Workspace : ToWorkspace  VariableName=PositionCmdFdbk  SaveFormat=Structure With Time  SampleTime=-1
  wires:
  Position Reference/1 -> Bus Selector1/1
  Bus Selector2/3 -> Mux/3  "<Z>"
  Bus Selector2/1 -> Mux/1  "<X>"
  Bus Selector1/1 -> Bus Creator/2
  Bus Creator/1 -> To Workspace/1
  Bus Selector2/2 -> Mux/2  "<Y>"
  Mux/1 -> Bus Creator/1
  Position Command/1 -> Bus Selector2/1

== system eVTOL_System/Flight Controller/Guidance Test Bench/Reference Tracking /Transition Reference ==
  States : Inport
  Bus Creator : BusCreator  Inputs=4
  Bus Selector4 : BusSelector  OutputSignals=airspeed,RotorParameters.Rotor A,Euler,Xe
  Gain : Gain  Gain=-1
  Selector : Selector  InputPortWidth=3  IndexOptions=Index vector (dialog)  Indices=[2]  OutputSizes=1
  Selector1 : Selector  InputPortWidth=3  IndexOptions=Index vector (dialog)  Indices=[3]  OutputSizes=1
  To Workspace1 : ToWorkspace  VariableName=TransitionFeedback  SaveFormat=Structure With Time  SampleTime=-1
  wires:
  States/1 -> Bus Selector4/1
  Bus Selector4/3 -> Selector/1  "<Euler>"
  Bus Selector4/4 -> Selector1/1  "<Xe>"
  Selector1/1 -> Gain/1
  Bus Selector4/1 -> Bus Creator/1  "<airspeed>"
  Selector/1 -> Bus Creator/3  "pitch"
  Gain/1 -> Bus Creator/4  "altitude"
  Bus Selector4/2 -> Bus Creator/2  "<Rotor A>"
  Bus Creator/1 -> To Workspace1/1

== system eVTOL_System/Motor Drive/Controller/Controller_HIL_CAN/CAN Communication 611 ==
  Speed_CMD_rpm : Inport
  Closed_loop : Inport  Port=2
  EnablePWM : Inport  Port=3
  Controller_Parameters : Inport  Port=4
  Bus Selector : BusSelector  OutputSignals=Ia_offset,Ib_offset,Kp_S,Ki_S,Kp_I,Ki_IxTcpu
  "CAN Read " : speedgoatlib_IO611/CAN Read   moduleType=IO611  id=1  channel=1  canType=CAN (HS)  useBusOut=on  HasMulRead=Specify by IDs  MsgIDlist=[1 2]  isEFF=off  LabelInHex=on  enableInput=off  ts=1e-3  initValues=[611 1 0.001 0 1 1 0 1 0 2 2 1 2]
      settings: LibrarySourceBlock=speedgoatlib_CANLIN_OfA2/CAN/CAN Read  SourceProductName=IO611
  CAN Unpack : canmsglib/CAN Unpack  MsgList=(none)  MsgName=Speed_TI_Out  MsgIDType=Standard (11-bit identifier)  MsgIdentifier=1  MsgLength=8  SignalInfo={ 'Speed_fbk', '0', '32', 'LE', 'single', 'Standard', '0', '1', '0', '-Inf', 'Inf'; 'Pos_fbk', '32', '32', 'LE', 'single', 'Standard', '0', '1', '0', '-Inf', 'Inf' }  IDPort=off  TimestampPort=off  ErrorPort=off  RemotePort=off  LengthPort=off  StatusPort=off  ApplyMinMax=off
      settings: LibrarySourceBlock=canlib/CAN Unpack
  CAN Unpack2 : canmsglib/CAN Unpack  MsgList=(none)  MsgName=Speed_Cmd_fbk  MsgIDType=Standard (11-bit identifier)  MsgIdentifier=2  MsgLength=8  SignalInfo={ 'Speed_Cmd', '0', '32', 'LE', 'single', 'Standard', '0', '1', '0', '-Inf', 'Inf'; 'Spd_pot', '32', '32', 'LE', 'single', 'Standard', '0', '1', '0', '-Inf', 'Inf' }  IDPort=off  TimestampPort=off  ErrorPort=off  RemotePort=off  LengthPort=off  StatusPort=off  ApplyMinMax=off
      settings: LibrarySourceBlock=canlib/CAN Unpack
  "CAN Write " : speedgoatlib_IO611/CAN Write   moduleType=IO611  id=1  channel=1  canType=CAN (HS)  useBusIn=on  numOfMsg=4  enableInput=on  enableStatusPort=off  initValues=[611 1 0.2 0 1 1 0 4 1 1]  ts=Ts_CAN_Tx
      settings: LibrarySourceBlock=speedgoatlib_CANLIN_OfA2/CAN/CAN Write  SourceProductName=IO611
  "CAN and LIN Setup " : speedgoatlib_IO611/CAN and LIN Setup   moduleInitValues="[611    1    1   -1   -1]"  id=1  moduleType=IO611  pciSlot=-1  canChn1=CAN (HS)  canChn2=Disabled  canChn3=Disabled  canChn4=Disabled  linChn1=Disabled  linChn2=Disabled  canInitStructArray=[]  canTermStructArray=[]  canChn1InitValues="[2   2   1  31   8   2   1   5   2]"  arbBdrChn1=1.0 MBaud  arbManBdrChn1=[2,1,31,8]  fdBdrChn1=5.0 MBaud  fdManBdrChn1=[2,1,5,2]  canChn2InitValues="[1  200    1   31    8    2    1    5    2]"  arbBdrChn2=10 kBaud  arbManBdrChn2=[200,1,31,8]  fdBdrChn2=5.0 MBaud  fdManBdrChn2=[2,1,5,2]  canChn3InitValues="[1   2   1  31   8   2   1   5   2]"  arbBdrChn3=1.0 MBaud  arbManBdrChn3=[2,1,31,8]  fdBdrChn3=5.0 MBaud  fdManBdrChn3=[2,1,5,2]  canChn4InitValues="[1   2   1  31   8   2   1   5   2]"  arbBdrChn4=1.0 MBaud  arbManBdrChn4=[2,1,31,8]  fdBdrChn4=5.0 MBaud  fdManBdrChn4=[2,1,5,2]  bdrLIN1=19200  linChn1InitValues="[1  19200]"  bdrLIN2=19200  linChn2InitValues="[1  19200]"
      settings: SourceProductName=IO611
  CANPack_ManualSignals : canmsglib/CAN Pack  MsgList=(none)  MsgName=Speed_Cmd  MsgIDType=Standard (11-bit identifier)  MsgIdentifier=0  CANIDInput=off  MsgLength=8  Remote=off  ApplyMinMax=off  BusOutput=on  SignalInfo={ 'Speed_Cmd', '0', '32', 'LE', 'single', 'Standard', '0', '1', '0', '-Inf', 'Inf'; 'Closed_loop', '32', '8', 'LE', 'unsigned', 'Standard', '0', '1', '0', '-Inf', 'Inf'; 'EnablePWM', '40', '8', 'LE', 'unsigned', 'Standard', '0', '1', '0', '-Inf', 'Inf'; 'Filler', '48', '16', 'LE', 'signed', 'Standard', '0', '1', '0', '-Inf', 'Inf' }
      settings: DataFormat=manually specified signals
  CANPack_ManualSignals1 : canmsglib/CAN Pack  MsgList=(none)  MsgName=Speed_Parameters  MsgIDType=Standard (11-bit identifier)  MsgIdentifier=31  CANIDInput=off  MsgLength=8  Remote=off  ApplyMinMax=off  BusOutput=on  SignalInfo={ 'Kp_S', '0', '32', 'LE', 'single', 'Standard', '0', '1', '0', '-Inf', 'Inf'; 'Ki_S', '32', '32', 'LE', 'single', 'Standard', '0', '1', '0', '-Inf', 'Inf' }
      settings: DataFormat=manually specified signals
  CANPack_ManualSignals2 : canmsglib/CAN Pack  MsgList=(none)  MsgName=I_Offsets  MsgIDType=Standard (11-bit identifier)  MsgIdentifier=30  CANIDInput=off  MsgLength=8  Remote=off  ApplyMinMax=off  BusOutput=on  SignalInfo={ 'Ia_offset', '0', '32', 'LE', 'single', 'Standard', '0', '1', '0', '-Inf', 'Inf'; 'Ib_offset', '32', '32', 'LE', 'single', 'Standard', '0', '1', '0', '-Inf', 'Inf' }
      settings: DataFormat=manually specified signals
  CANPack_ManualSignals3 : canmsglib/CAN Pack  MsgList=(none)  MsgName=I_Parameters  MsgIDType=Standard (11-bit identifier)  MsgIdentifier=29  CANIDInput=off  MsgLength=8  Remote=off  ApplyMinMax=off  BusOutput=on  SignalInfo={ 'Kp_I', '0', '32', 'LE', 'single', 'Standard', '0', '1', '0', '-Inf', 'Inf'; 'Ki_I', '32', '32', 'LE', 'single', 'Standard', '0', '1', '0', '-Inf', 'Inf' }
      settings: DataFormat=manually specified signals
  Data Type Conversion : DataTypeConversion  OutDataTypeStr=boolean  SaturateOnIntegerOverflow=off  RndMeth=Floor
  Gain{,1..3} (4 alike) : Gain
  Mux : Mux
  Pulse Generator : DiscretePulseGenerator  Period=40  PulseWidth=10  SampleTime=Ts_CAN_Tx/10
  Pulse Generator1 : DiscretePulseGenerator  Period=40  PulseWidth=10  PhaseDelay=10  SampleTime=Ts_CAN_Tx/10
  Pulse Generator2 : DiscretePulseGenerator  Period=40  PulseWidth=10  PhaseDelay=20  SampleTime=Ts_CAN_Tx/10
  Pulse Generator3 : DiscretePulseGenerator  Period=40  PulseWidth=10  PhaseDelay=30  SampleTime=Ts_CAN_Tx/10
  Rate Transition{,1..3,5..9} (9 alike) : RateTransition  Integrity=off  Deterministic=off
  Rate Transition4 : RateTransition  Integrity=off  OutPortSampleTime=Ts_CAN_Tx
  Vector Concatenate : Concatenate  NumInputs=4
  Speed_fbk : Outport
  Pos_fdk : Outport  Port=2
  Speed_Cmd : Outport  Port=3
  Spd_pot : Outport  Port=4
  wires:
  "CAN Read "/2 -> CAN Unpack/1
  CAN Unpack/1 -> Speed_fbk/1
  CAN Unpack/2 -> Pos_fdk/1
  "CAN Read "/3 -> CAN Unpack2/1
  CAN Unpack2/2 -> Spd_pot/1
  CAN Unpack2/1 -> Speed_Cmd/1
  Bus Selector/3 -> Rate Transition6/1  "<Kp_S>"
  Bus Selector/4 -> Rate Transition5/1  "<Ki_S>"
  Bus Selector/2 -> Rate Transition1/1  "<Ib_offset>"
  Bus Selector/1 -> Rate Transition/1  "<Ia_offset>"
  Controller_Parameters/1 -> Bus Selector/1
  Bus Selector/6 -> Rate Transition2/1  "<Ki_IxTcpu>"
  Bus Selector/5 -> Rate Transition3/1  "<Kp_I>"
  CANPack_ManualSignals1/1 -> Vector Concatenate/3  "CAN_Ch1_ID102_Tx"
  CANPack_ManualSignals2/1 -> Vector Concatenate/2  "CAN_Ch1_ID102_Tx"
  Pulse Generator/1 -> Gain3/1
  CANPack_ManualSignals/1 -> Vector Concatenate/1  "CAN_Ch1_ID102_Tx"
  Data Type Conversion/1 -> Rate Transition4/1
  Pulse Generator2/1 -> Gain1/1
  Pulse Generator1/1 -> Gain/1
  Mux/1 -> Data Type Conversion/1
  CANPack_ManualSignals3/1 -> Vector Concatenate/4  "CAN_Ch1_ID102_Tx"
  Pulse Generator3/1 -> Gain2/1
  Rate Transition/1 -> CANPack_ManualSignals2/1
  Rate Transition1/1 -> CANPack_ManualSignals2/2
  Rate Transition6/1 -> CANPack_ManualSignals1/1
  Rate Transition5/1 -> CANPack_ManualSignals1/2
  Rate Transition3/1 -> CANPack_ManualSignals3/1
  Rate Transition2/1 -> CANPack_ManualSignals3/2
  Speed_CMD_rpm/1 -> Rate Transition7/1
  Rate Transition7/1 -> CANPack_ManualSignals/1
  Closed_loop/1 -> Rate Transition8/1
  Rate Transition8/1 -> CANPack_ManualSignals/2
  EnablePWM/1 -> Rate Transition9/1
  Rate Transition9/1 -> CANPack_ManualSignals/3
  Gain3/1 -> Mux/1
  Gain/1 -> Mux/2
  Gain1/1 -> Mux/3
  Gain2/1 -> Mux/4
  Vector Concatenate/1 -> "CAN Write "/2
  Rate Transition4/1 -> "CAN Write "/1

== system eVTOL_System/Motor Drive/Controller/Controller_HIL_CAN/Internal PWM configuration1 ==
  Bus Creator1 : BusCreator  Inputs=5
  Not Used Dc : Constant  Value=[0 0 0]  OutDataTypeStr=double
  Not Used Period : Constant  Value=[1 1 1]  OutDataTypeStr=double
  PWM Generation : pwm_cpulib/PWM Generation  f_FPGA=f_FPGA  n_channels=3  sel_scaling=CPU  protection_param=A/B are forced off when A/B are on.  deadband_sec=0  natural_update=At period starts  delay=0  trigger_duration_sec=[1e-6]  trigger_period_start=on  trigger_half_of_the_period=off  trigger_a_on=off  trigger_a_off=off  trigger_b_on=off  trigger_b_off=off  bit_width_pwm_gen=24  invert_a=off  invert_b=on  invert_c=off  showPhaseInput=off
      settings: SourceProductName=PWM CPU Library
  bias4 : Constant  Value=0  OutDataTypeStr=boolean  SampleTime=Ts_UI
  bias5 : Constant  Value=0  OutDataTypeStr=boolean  SampleTime=Ts_UI
  bias6 : Constant  OutDataTypeStr=boolean  SampleTime=Ts_UI
  Simu Config : Outport
  wires:
  PWM Generation/2 -> Bus Creator1/3  "PCIe_PWM_Runtime"
  bias6/1 -> Bus Creator1/5  "PCIe_Protocol"
  PWM Generation/1 -> Bus Creator1/2  "PCIe_PWM_Config"
  Bus Creator1/1 -> Simu Config/1
  bias4/1 -> Bus Creator1/1  "PCIe_RC_or_TTL"
  bias5/1 -> Bus Creator1/4  "PCIe_PWM_Enable"
  Not Used Period/1 -> PWM Generation/1
  Not Used Dc/1 -> PWM Generation/2

== system eVTOL_System/Motor Drive/Controller/Controller_MIL/F28379D ADC ==
  Iab_IO334V : Inport
  Add Constant : Bias  Bias=Ia_offset  SaturateOnIntegerOverflow=off
  Add Constant1 : Bias  Bias=Ib_offset  SaturateOnIntegerOverflow=off
  Demux : Demux  Outputs=2
  Gain : Gain  Gain=2^12/F28379D_ADC_Vmax
  Ia_ADC : Outport
  Ib_ADC : Outport  Port=2
  wires:
  Iab_IO334V/1 -> Gain/1
  Gain/1 -> Demux/1
  Demux/1 -> Add Constant/1
  Demux/2 -> Add Constant1/1
  Add Constant/1 -> Ia_ADC/1
  Add Constant1/1 -> Ib_ADC/1
